simulink model "Modelo2Simulink"  (R2021a)
settings: Solver=FixedStepAuto  StartTime=0.0  StopTime=20000  FixedStep=1e-3  RelTol=1e-3
settings Model: Creator=User  LastModifiedBy=User

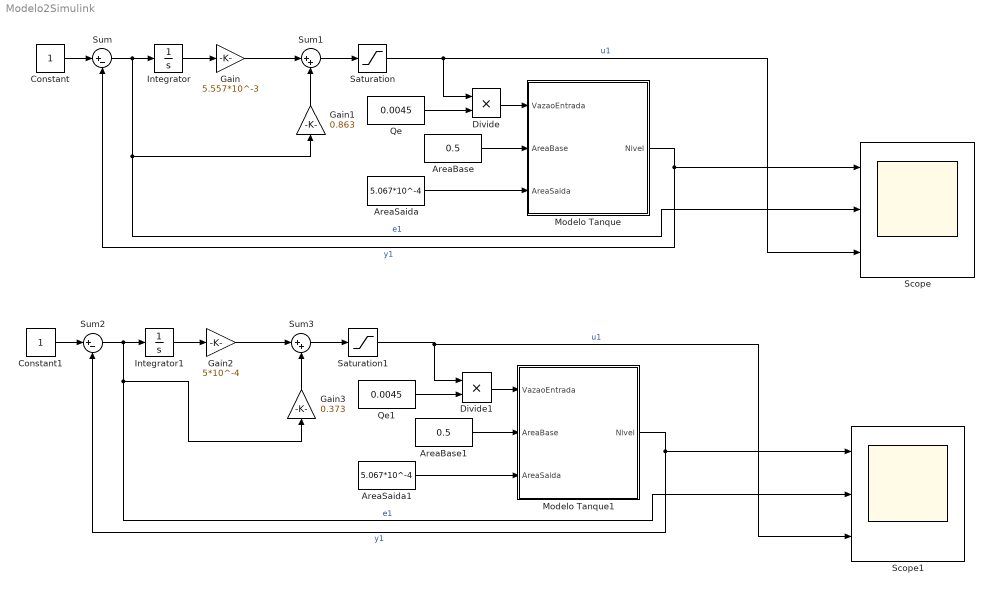
== system Modelo2Simulink ==
  AreaBase : Constant  Value=0.5
  AreaBase1 : Constant  Value=0.5
  AreaSaida : Constant  Value=5.067*10^-4
  AreaSaida1 : Constant  Value=5.067*10^-4
  Constant : Constant
  Constant1 : Constant
  Divide : Product  Inputs=**
  Divide1 : Product  Inputs=**
  Gain : Gain  Gain=5.557*10^-3
  Gain1 : Gain  Gain=0.863
  Gain2 : Gain  Gain=5*10^-4
  Gain3 : Gain  Gain=0.373
  Integrator : Integrator
  Integrator1 : Integrator
  Modelo Tanque : Subsystem
  Modelo Tanque1 : Subsystem
  Qe : Constant  Value=0.0045
  Qe1 : Constant  Value=0.0045
  Saturation : Saturate  UpperLimit=1  LowerLimit=0
  Saturation1 : Saturate  UpperLimit=1  LowerLimit=0
  Scope : Scope  NumInputPorts=3
  Scope1 : Scope  NumInputPorts=3
  Sum : Sum  Inputs=|+-
  Sum1 : Sum  Inputs=|++
  Sum2 : Sum  Inputs=|+-
  Sum3 : Sum  Inputs=|++
  wires:
  AreaBase/1 -> Modelo Tanque/2(AreaBase)
  AreaSaida/1 -> Modelo Tanque/3(AreaSaida)
  Modelo Tanque/1(Nivel) -> Sum/2, Scope/1  "y1"
  Qe/1 -> Divide/2
  Divide/1 -> Modelo Tanque/1(VazaoEntrada)
  Constant/1 -> Sum/1
  Integrator/1 -> Gain/1
  Gain/1 -> Sum1/1
  Gain1/1 -> Sum1/2
  Saturation/1 -> Divide/1, Scope/3  "u1"
  Sum/1 -> Integrator/1, Gain1/1, Scope/2  "e1"
  Sum1/1 -> Saturation/1
  Sum3/1 -> Saturation1/1
  Sum2/1 -> Gain3/1, Scope1/2, Integrator1/1  "e1"
  Saturation1/1 -> Scope1/3, Divide1/1  "u1"
  Gain3/1 -> Sum3/2
  Gain2/1 -> Sum3/1
  Integrator1/1 -> Gain2/1
  Constant1/1 -> Sum2/1
  Divide1/1 -> Modelo Tanque1/1(VazaoEntrada)
  Qe1/1 -> Divide1/2
  Modelo Tanque1/1(Nivel) -> Scope1/1, Sum2/2  "y1"
  AreaSaida1/1 -> Modelo Tanque1/3(AreaSaida)
  AreaBase1/1 -> Modelo Tanque1/2(AreaBase)

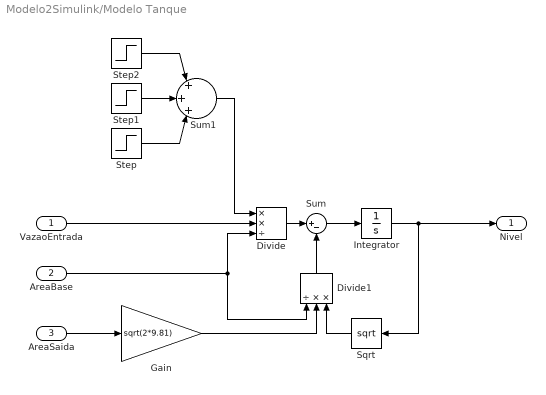
== system Modelo2Simulink/Modelo Tanque ==
  VazaoEntrada : Inport
  AreaBase : Inport  Port=2
  AreaSaida : Inport  Port=3
  Divide : Product  Inputs=**/
  Divide1 : Product  Inputs=/**
  Gain : Gain  Gain=sqrt(2*9.81)
  Integrator : Integrator
  Sqrt : Sqrt  SaturateOnIntegerOverflow=on
  Step : Step  Time=1500  Before=1/3  After=1/6  SampleTime=0
  Step1 : Step  Time=3000  Before=1/3  After=1/6  SampleTime=0
  Step2 : Step  Time=5000  Before=1/3  After=2/3  SampleTime=0
  Sum : Sum  Inputs=|+-
  Sum1 : Sum  Inputs=|+|+|+|
  Nivel : Outport
  wires:
  Sqrt/1 -> Divide1/3
  AreaBase/1 -> Divide1/1, Divide/3
  Integrator/1 -> Nivel/1, Sqrt/1
  Sum/1 -> Integrator/1
  VazaoEntrada/1 -> Divide/2
  Divide1/1 -> Sum/2
  Divide/1 -> Sum/1
  AreaSaida/1 -> Gain/1
  Gain/1 -> Divide1/2
  Step/1 -> Sum1/3
  Step1/1 -> Sum1/2
  Step2/1 -> Sum1/1
  Sum1/1 -> Divide/1

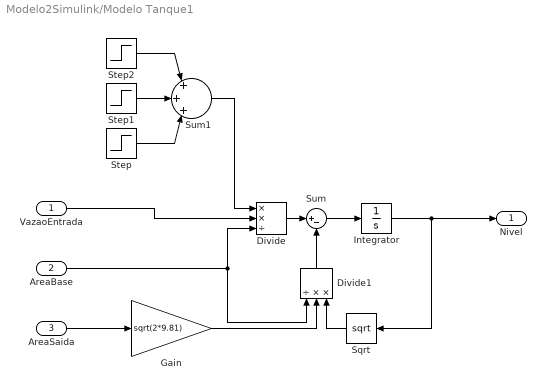
== system Modelo2Simulink/Modelo Tanque1 ==
  VazaoEntrada : Inport
  AreaBase : Inport  Port=2
  AreaSaida : Inport  Port=3
  Divide : Product  Inputs=**/
  Divide1 : Product  Inputs=/**
  Gain : Gain  Gain=sqrt(2*9.81)
  Integrator : Integrator
  Sqrt : Sqrt  SaturateOnIntegerOverflow=on
  Step : Step  Time=6000  Before=1/3  After=1/6  SampleTime=0
  Step1 : Step  Time=9500  Before=1/3  After=1/6  SampleTime=0
  Step2 : Step  Time=12500  Before=1/3  After=2/3  SampleTime=0
  Sum : Sum  Inputs=|+-
  Sum1 : Sum  Inputs=|+|+|+|
  Nivel : Outport
  wires:
  Gain/1 -> Divide1/2
  AreaSaida/1 -> Gain/1
  Divide/1 -> Sum/1
  Divide1/1 -> Sum/2
  VazaoEntrada/1 -> Divide/2
  Sum/1 -> Integrator/1
  Integrator/1 -> Sqrt/1, Nivel/1
  AreaBase/1 -> Divide/3, Divide1/1
  Sqrt/1 -> Divide1/3
  Sum1/1 -> Divide/1
  Step/1 -> Sum1/3
  Step1/1 -> Sum1/2
  Step2/1 -> Sum1/1
